simulink model "APP"  (R2016b)
settings: Solver=VariableStepAuto  StartTime=0.0  StopTime=10.0  RelTol=1e-3
settings Model: Creator=wangrui  LastModifiedBy=guanxiaoxing

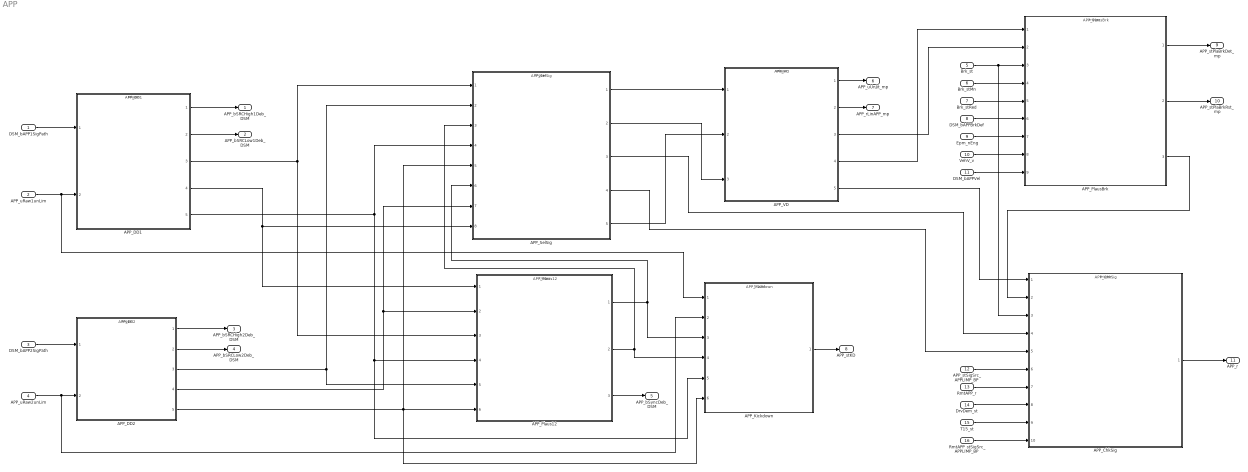
== system APP ==
  DSM_bAPP1SigPath : Inport  Description=status of FId_APP1SigPath  OutMin=0  OutMax=1  OutDataTypeStr=boolean
  APP_uRaw1unLim : Inport  Tag=mv  Description=Acceleration pedal sensor 1 unlimited raw value  Port=2  OutMin=0  OutMax=5000  OutDataTypeStr=Ad_mv
  DSM_bAPP2SigPath : Inport  Description=status of FId_APP2SigPath  Port=3  OutMin=0  OutMax=1  OutDataTypeStr=boolean
  APP_uRaw2unLim : Inport  Tag=mv  Description=Acceleration pedal sensor 2 unlimited raw value  Port=4  OutMin=0  OutMax=5000  OutDataTypeStr=Ad_mv
  Brk_st : Inport  Description=Brake switch state  Port=5  OutMin=0  OutMax=255  OutDataTypeStr=State_uint8
  Brk_stMn : Inport  Description=Status of the main brake  Port=6  OutMin=0  OutMax=1  OutDataTypeStr=boolean
  Brk_stRed : Inport  Description=Status of the redundant break  Port=7  OutMin=0  OutMax=1  OutDataTypeStr=boolean
  DSM_bAPPBrkDef : Inport  Description=status of FId_APPBrkDef  Port=8  OutMin=0  OutMax=1  OutDataTypeStr=boolean
  Epm_nEng : Inport  Tag=rpm  Description=Engine speed  Port=9  OutMin=0  OutMax=6000  OutDataTypeStr=EngSpeed_rpm
  VehV_v : Inport  Tag=km/h  Description=Vehicle speed  Port=10  OutMin=0  OutMax=250  OutDataTypeStr=VehSpeed_km_h
  DSM_bAPPVel : Inport  Description=status of FId_APPVel  Port=11  OutMin=0  OutMax=1  OutDataTypeStr=boolean
  APP_stSigSrc_APPLIMP_BP : Inport  Description=Substitute operation active, accelerator pedal sensor value and accelerator pedal sensor increase are limited  Port=12  OutMin=0  OutMax=1  OutDataTypeStr=boolean
  RmtAPP_r : Inport  Tag=%  Description=Value of Remote accelerator pedal Position  Port=13  OutMin=0  OutMax=100  OutDataTypeStr=Accpedal_rate
  DrvDem_st : Inport  Description=Drive demand status to select the pedal for setpoint calculation  Port=14  OutMin=0  OutMax=255  OutDataTypeStr=State_uint8
  T15_st : Inport  Description=Terminal 15 status after debouncing  Port=15  OutDataTypeStr=Enum: Switch_conv
  RmtAPP_stSigSrc_APPLIMP_BP : Inport  Description=Substitute operation active, remote accelerator pedal sensor value and accelerator pedal sensor increase are limited  Port=16  OutMin=0  OutMax=1  OutDataTypeStr=boolean
  APP_ChkSig : ModelReference  ModelNameDialog=APP_ChkSig  SimulationMode=Normal  ModelReferenceVersion=1.57  TriggerPortName=function  TriggerPortTriggerType=function-call  TriggerPortStatesWhenEnabling=held
  APP_DD1 : ModelReference  ModelNameDialog=APP_DD1  SimulationMode=Normal  ModelReferenceVersion=1.20  TriggerPortName=function  TriggerPortTriggerType=function-call  TriggerPortStatesWhenEnabling=held
  APP_DD2 : ModelReference  ModelNameDialog=APP_DD2  SimulationMode=Normal  ModelReferenceVersion=1.14  TriggerPortName=function  TriggerPortTriggerType=function-call  TriggerPortStatesWhenEnabling=held
  APP_Kickdown : ModelReference  ModelNameDialog=APP_Kickdown  SimulationMode=Normal  ModelReferenceVersion=1.8  TriggerPortName=function  TriggerPortTriggerType=function-call  TriggerPortStatesWhenEnabling=held
  APP_Plaus12 : ModelReference  ModelNameDialog=APP_Plaus12  SimulationMode=Normal  ModelReferenceVersion=1.24  TriggerPortName=function  TriggerPortTriggerType=function-call  TriggerPortStatesWhenEnabling=held
  APP_PlausBrk : ModelReference  ModelNameDialog=APP_PlausBrk  SimulationMode=Normal  ModelReferenceVersion=1.27  TriggerPortName=function  TriggerPortTriggerType=function-call  TriggerPortStatesWhenEnabling=held
  APP_SelSig : ModelReference  ModelNameDialog=APP_SelSig  SimulationMode=Normal  ModelReferenceVersion=1.26  TriggerPortName=function  TriggerPortTriggerType=function-call  TriggerPortStatesWhenEnabling=held
  APP_VD : ModelReference  ModelNameDialog=APP_VD  SimulationMode=Normal  ModelReferenceVersion=1.35  TriggerPortName=function  TriggerPortTriggerType=function-call  TriggerPortStatesWhenEnabling=held
  APP_bSRCHigh1Deb_DSM : Outport  Description=Status debounced SRC-High error Sensor 1  OutMin=0  OutMax=1  OutDataTypeStr=boolean
  APP_bSRCLow1Deb_DSM : Outport  Description=Status debounced SRC-Low error Sensor 1  Port=2  OutMin=0  OutMax=1  OutDataTypeStr=boolean
  APP_bSRCHigh2Deb_DSM : Outport  Description=Status debounced SRC-High error Sensor 2  Port=3  OutMin=0  OutMax=1  OutDataTypeStr=boolean
  APP_bSRCLow2Deb_DSM : Outport  Description=Status debounced SRC-Low error Sensor 2  Port=4  OutMin=0  OutMax=1  OutDataTypeStr=boolean
  APP_bSyncDeb_DSM : Outport  Description=Status debounced sync check finally defect  Port=5  OutMin=0  OutMax=1  OutDataTypeStr=boolean
  APP_uUnJit_mp : Outport  Tag=mv  Description=Acceleration pedal position unjittered value  Port=6  OutMin=0  OutMax=5000  OutDataTypeStr=Ad_mv
  APP_rLinAPP_mp : Outport  Tag=%  Description=Linearisation ratio of accelerator pedal  Port=7  OutMin=0  OutMax=100  OutDataTypeStr=Accpedal_rate
  APP_stKD : Outport  Description=State of accelerator pedal kick down  Port=8  OutMin=0  OutMax=1  OutDataTypeStr=boolean
  APP_stPlaBrkDet_mp : Outport  Description=State of detection plausibility with brake  Port=9  OutMin=0  OutMax=1  OutDataTypeStr=boolean
  APP_stPlaBrkRst_mp : Outport  Description=State of reset plausibility with brake  Port=10  OutMin=0  OutMax=1  OutDataTypeStr=boolean
  APP_r : Outport  Tag=%  Description=Acceleration pedal sensor 1 value after fault handling  Port=11  OutMin=0  OutMax=100  OutDataTypeStr=Accpedal_rate
  wires:
  DSM_bAPP1SigPath/1 -> APP_DD1/1
  DSM_bAPP2SigPath/1 -> APP_DD2/1
  APP_DD1/1 -> APP_bSRCHigh1Deb_DSM/1
  APP_DD1/2 -> APP_bSRCLow1Deb_DSM/1
  APP_DD2/1 -> APP_bSRCHigh2Deb_DSM/1
  APP_DD2/2 -> APP_bSRCLow2Deb_DSM/1
  APP_DD2/4 -> APP_SelSig/7, APP_Plaus12/2
  APP_DD1/3 -> APP_Plaus12/3, APP_SelSig/1
  APP_DD1/4 -> APP_Plaus12/1, APP_SelSig/8
  APP_DD2/3 -> APP_SelSig/2, APP_Plaus12/5
  APP_Plaus12/3 -> APP_bSyncDeb_DSM/1
  APP_SelSig/1 -> APP_VD/1
  APP_SelSig/5 -> APP_VD/2
  APP_SelSig/2 -> APP_VD/3
  APP_uRaw1unLim/1 -> APP_Kickdown/1, APP_DD1/2
  APP_uRaw2unLim/1 -> APP_Kickdown/2, APP_DD2/2
  APP_Plaus12/2 -> APP_Kickdown/4, APP_SelSig/3
  APP_Plaus12/1 -> APP_Kickdown/3, APP_SelSig/6
  APP_DD1/5 -> APP_Plaus12/4, APP_Kickdown/5, APP_SelSig/4
  APP_DD2/5 -> APP_Kickdown/6, APP_SelSig/5, APP_Plaus12/6
  APP_VD/1 -> APP_uUnJit_mp/1
  APP_VD/2 -> APP_rLinAPP_mp/1
  APP_Kickdown/1 -> APP_stKD/1
  DSM_bAPPVel/1 -> APP_PlausBrk/9
  APP_VD/4 -> APP_PlausBrk/1
  APP_VD/3 -> APP_PlausBrk/2
  Brk_stMn/1 -> APP_PlausBrk/4
  Brk_stRed/1 -> APP_PlausBrk/5
  DSM_bAPPBrkDef/1 -> APP_PlausBrk/6
  Epm_nEng/1 -> APP_PlausBrk/7
  VehV_v/1 -> APP_PlausBrk/8
  APP_PlausBrk/1 -> APP_stPlaBrkDet_mp/1
  APP_PlausBrk/2 -> APP_stPlaBrkRst_mp/1
  APP_ChkSig/1 -> APP_r/1
  RmtAPP_r/1 -> APP_ChkSig/7
  T15_st/1 -> APP_ChkSig/9
  DrvDem_st/1 -> APP_ChkSig/8
  RmtAPP_stSigSrc_APPLIMP_BP/1 -> APP_ChkSig/10
  APP_VD/5 -> APP_ChkSig/1
  APP_PlausBrk/3 -> APP_ChkSig/2
  Brk_st/1 -> APP_PlausBrk/3, APP_ChkSig/3
  APP_stSigSrc_APPLIMP_BP/1 -> APP_ChkSig/6
  APP_SelSig/4 -> APP_ChkSig/5
  APP_SelSig/3 -> APP_ChkSig/4
